simulink model "Model_6DOF_dk"  (R2022a)
settings: Solver=FixedStepAuto  StartTime=0.0  StopTime=Tf  FixedStep=0.05  RelTol=1e-3
InitFcn:
  | run;
StopFcn:
  | save('testdata')
values from neighbouring files (symbols this model uses):
  adap = 1    [run.m]    (also in testdata.mat)
  Ba_0 = [0 0 0 0 0 0]    [run.m]    (also in testdata.mat)
  Bb = 4418825.3321    [testdata.mat]
  Bv_0 = [-5.14444 0 0 0 0 0]    [run.m]    (also in testdata.mat)
  Bx_0 = [0 0 -12 0 0 0]    [run.m]    (also in testdata.mat)
  dA_BP1 = [0.00388591051125 0.00354364911083 0.00553040741788 0.00502167988714 0.0078585088908 0.00748424955325 0.0119232766011 0.0109054787122 0.0168329706434 0.016985509009 0.0156802934897 0.014556760782 ... (616 elements, 616x1)]    [testdata.mat]
  dA_BP2 = [0.00388594063171 0.00354357191533 0.00553040491113 0.00502170939051 0.00785855989083 0.00748435285791 0.0119232653011 0.0109054419481 0.0168329955973 0.0169854794658 0.015680230324 0.0145567225609 ... (616 elements, 616x1)]    [testdata.mat]
  dA_Hull = [0.896301676511 0.898896720864 0.884294141897 0.886832830172 0.870887902011 0.873360353662 0.856223658523 0.858613244346 0.840314828191 0.842595287849 0.823129385532 0.8253007603 ... (2914 elements, 2914x1)]    [testdata.mat]
  dA_PH = [0.00917454029683 0.00917454029683 0.00646521761836 0.00644666811643 0.011728531678 0.0107683420972 0.0165186720105 0.0100399866209 0.0121147162203 0.00917369783051 0.00917369783051 0.00646462373197 ... (550 elements, 550x1)]    [testdata.mat]
  dA_Sail = [0.08073747293 0.0655437895785 0.0678199581962 0.211496702297 0.185444652254 0.10949647106 0.0763960001413 0.0735864235671 0.0440728222699 0.281106392154 0.32735958292 0.104041938486 ... (564 elements, 564x1)]    [testdata.mat]
  dA_SProot = [0.0225345452169 0.0247277274893 0.0225345452169 0.0480467976325 0.0166447079844 0.0410754287554 0.0247277274893 0.0480467976325 0.0468898715351 0.0839833312794 0.0166447079844 0.0255016718 ... (904 elements, 904x1)]    [testdata.mat]
  dA_X1a = [0.0149621011817 0.0166706156701 0.0341149781095 0.0355915100668 0.0512235531199 0.0489176133683 0.0604458424392 0.0503279152264 0.0577124835488 0.0401555322121 0.044833653096 0.0251568218541 ... (200 elements, 200x1)]    [testdata.mat]
  dA_X1b = [0.0149621011817 0.0166706156701 0.0341149781095 0.0355915100668 0.0512235531199 0.0489176133683 0.0604458424392 0.0503279152264 0.0577124835488 0.0401555322121 0.044833653096 0.0251568218541 ... (200 elements, 200x1)]    [testdata.mat]
  dA_X2a = [0.0149620639393 0.0166705502855 0.0341150948266 0.0355913495849 0.051223110376 0.0489180393921 0.0604458270347 0.0503275686692 0.0577128112225 0.0401556683139 0.0448334591683 0.0251566482124 ... (200 elements, 200x1)]    [testdata.mat]
  dA_X2b = [0.0149620639393 0.0166705502855 0.0341150948266 0.0355913495849 0.051223110376 0.0489180393921 0.0604458270347 0.0503275686692 0.0577128112225 0.0401556683139 0.0448334591683 0.0251566482124 ... (200 elements, 200x1)]    [testdata.mat]
  dA_X3a = [0.0149621011817 0.0166706156701 0.0341149781095 0.0355915100668 0.0512235531199 0.0489176133683 0.0604458424392 0.0503279152264 0.0577124835488 0.0401555322121 0.044833653096 0.0251568218541 ... (200 elements, 200x1)]    [testdata.mat]
  dA_X3b = [0.0149621011817 0.0166706156701 0.0341149781095 0.0355915100668 0.0512235531199 0.0489176133683 0.0604458424392 0.0503279152264 0.0577124835488 0.0401555322121 0.044833653096 0.0251568218541 ... (200 elements, 200x1)]    [testdata.mat]
  dA_X4a = [0.0149621011817 0.0166706156701 0.0341149781095 0.0355915100668 0.0512235531199 0.0489176133683 0.0604458424392 0.0503279152264 0.0577124835488 0.0401555322121 0.044833653096 0.0251568218541 ... (200 elements, 200x1)]    [testdata.mat]
  dA_X4b = [0.0149621011817 0.0166706156701 0.0341149781095 0.0355915100668 0.0512235531199 0.0489176133683 0.0604458424392 0.0503279152264 0.0577124835488 0.0401555322121 0.044833653096 0.0251568218541 ... (200 elements, 200x1)]    [testdata.mat]
  Ixx = 52300000    [testdata.mat]
  Ixy = 0    [testdata.mat]
  Ixz = 0    [testdata.mat]
  Iyy = 1375000000    [testdata.mat]
  Iyz = 0    [testdata.mat]
  Izz = 1367000000    [testdata.mat]
  L1 =     [testdata.mat]
  Mb = 4418825.3321    [testdata.mat]
  n_BP1 = [-0.7747315 -0.03638153 -0.4095958 0 -0.1221389 0 -0.01670914 0 0.005209626 0 0.03404154 0 ... (1848 elements, 616x3)]    [testdata.mat]
  n_BP2 = [-0.774731517 -0.0363815315 -0.409595788 0 -0.122138903 0 -0.0167091396 0 0.00520962616 0 0.0340415388 0 ... (1848 elements, 616x3)]    [testdata.mat]
  n_Hull = [-3.334458e-05 -1.700098e-14 -3.354233e-05 -1.686235e-14 -3.289162e-05 -1.685701e-14 -3.291391e-05 -1.698144e-14 -3.338145e-05 -1.688959e-14 -3.29289e-05 -1.682536e-14 ... (8742 elements, 2914x3)]    [testdata.mat]
  n_PH = [0 0 0.01711651 0.01711627 0.2676807 0.2676804 0.7675173 0.7675174 0.9857236 0 0 0.01711456 ... (1650 elements, 550x3)]    [testdata.mat]
  n_Sail = [-0.05126832 -0.05168081 -0.0485872 -0.03288998 -0.03203588 -0.04435105 -0.04335441 -0.04419429 -0.05169604 0.01094904 0.01649325 -0.03825178 ... (1692 elements, 564x3)]    [testdata.mat]
  n_SProot = [-0.7837688 -0.7969784 -0.7837688 -0.79448 -0.280412 -0.3378876 -0.7969784 -0.79448 -0.7910827 -0.3483897 -0.280412 -0.2790298 ... (2712 elements, 904x3)]    [testdata.mat]
  n_X2a = [-0.283297986 -0.283136904 -0.283195704 -0.28313759 -0.2831586 -0.283137113 -0.28313911 -0.283136606 -0.283121586 -0.283136815 -0.283108413 -0.283138901 ... (600 elements, 200x3)]    [testdata.mat]
  n_X2b = [-0.283297986 -0.283136904 -0.283195704 -0.28313759 -0.2831586 -0.283137113 -0.28313911 -0.283136606 -0.283121586 -0.283136815 -0.283108413 -0.283138901 ... (600 elements, 200x3)]    [testdata.mat]
  n_X3a = [-0.283298 -0.2831369 -0.2831957 -0.2831376 -0.2831586 -0.2831371 -0.2831391 -0.2831366 -0.2831216 -0.2831368 -0.2831084 -0.2831389 ... (600 elements, 200x3)]    [testdata.mat]
  n_X4a = [-0.283298 -0.2831369 -0.2831957 -0.2831376 -0.2831586 -0.2831371 -0.2831391 -0.2831366 -0.2831216 -0.2831368 -0.2831084 -0.2831389 ... (600 elements, 200x3)]    [testdata.mat]
  n_X4b = [-0.283298 -0.2831369 -0.2831957 -0.2831376 -0.2831586 -0.2831371 -0.2831391 -0.2831366 -0.2831216 -0.2831368 -0.2831084 -0.2831389 ... (600 elements, 200x3)]    [testdata.mat]
  nt_BP1 = 616    [testdata.mat]
  nt_BP2 = 616    [testdata.mat]
  nt_Hull = 2914    [testdata.mat]
  nt_PH = 550    [testdata.mat]
  nt_Sail = 564    [testdata.mat]
  nt_SProot = 904    [testdata.mat]
  nt_X1a = 200    [testdata.mat]
  nt_X1b = 200    [testdata.mat]
  nt_X2a = 200    [testdata.mat]
  nt_X2b = 200    [testdata.mat]
  nt_X3a = 200    [testdata.mat]
  nt_X3b = 200    [testdata.mat]
  nt_X4a = 200    [testdata.mat]
  nt_X4b = 200    [testdata.mat]
  psi_ref = 0    [run.m]    (also in testdata.mat)
  Seastate = 0    [run.m]    (also in testdata.mat)
  Ts = 0.05    [run.m]    (also in testdata.mat)
  v_ref = Bv_0(1)    [run.m]    (also in testdata.mat = -5.14444)
  vt1_BP1 = [-11.0524049722 -10.9924120522 -10.9924120522 -10.8819663922 -10.8819663922 -10.7297166322 -10.7297166322 -10.5070632922 -10.5070632922 -10.1807245522 -10.1807245522 -9.8815181122 ... (1848 elements, 616x3)]    [testdata.mat]
  vt1_BP2 = [-11.0524048318 -10.9924111396 -10.9924111396 -10.8819658306 -10.8819658306 -10.7297157898 -10.7297157898 -10.5070637134 -10.5070637134 -10.1807238502 -10.1807238502 -9.8815188844 ... (1848 elements, 616x3)]    [testdata.mat]
  vt1_Hull = [3.5122487678 3.7304022878 5.2621803278 5.4863499878 6.9866994878 7.2167238278 8.6832650078 8.9189474678 10.3493567078 10.5904445678 11.9823842078 12.2286247478 ... (8742 elements, 2914x3)]    [testdata.mat]
  vt1_PH = [37.3342788278 37.3342788278 37.4268866678 37.4268866678 37.5892452278 37.5892452278 37.7549453078 37.7549453078 37.8074619278 37.3342788278 37.3342788278 37.4268866678 ... (1650 elements, 550x3)]    [testdata.mat]
  vt1_Sail = [-12.4909433722 -12.1578443722 -12.0399645322 -11.2138368922 -10.6240515922 -11.5111900522 -11.9364967522 -11.6561249722 -12.4909433722 -7.5732648922 -6.8453119522 -11.1890071522 ... (1692 elements, 564x3)]    [testdata.mat]
  vt1_SProot = [29.2099766678 29.1371231078 29.0494854278 29.2099766678 29.2862630078 29.4526510478 29.0494854278 29.1261368078 29.3369263478 29.5706712878 29.0494854278 29.3857364078 ... (2712 elements, 904x3)]    [testdata.mat]
  vt1_X1a = [29.3961751478 29.4776282078 29.4776282078 29.7060309278 29.7060309278 30.0693861278 30.0693861278 30.5458756478 30.5458756478 31.0830460478 31.0830460478 31.6023926678 ... (600 elements, 200x3)]    [testdata.mat]
  vt1_X1b = [29.6638337078 29.6638337078 29.9620713878 29.9620713878 30.3181187678 30.3181187678 30.7116389078 30.7116389078 31.1104380878 31.1104380878 31.4810519678 31.4810519678 ... (600 elements, 200x3)]    [testdata.mat]
  vt1_X2a = [29.3961767624 29.4776272952 29.4776272952 29.7060326828 29.7060326828 30.0693842324 30.0693842324 30.5458736822 30.5458736822 31.083047171 31.083047171 31.6023916148 ... (600 elements, 200x3)]    [testdata.mat]
  vt1_X2b = [29.6638345502 29.6638345502 29.9620708964 29.9620708964 30.3181168022 30.3181168022 30.7116409436 30.7116409436 31.1104372454 31.1104372454 31.4810526698 31.4810526698 ... (600 elements, 200x3)]    [testdata.mat]
  vt1_X3a = [29.3961751478 29.4776282078 29.4776282078 29.7060309278 29.7060309278 30.0693861278 30.0693861278 30.5458756478 30.5458756478 31.0830460478 31.0830460478 31.6023926678 ... (600 elements, 200x3)]    [testdata.mat]
  vt1_X3b = [29.6638337078 29.6638337078 29.9620713878 29.9620713878 30.3181187678 30.3181187678 30.7116389078 30.7116389078 31.1104380878 31.1104380878 31.4810519678 31.4810519678 ... (600 elements, 200x3)]    [testdata.mat]
  vt1_X4a = [29.6638337078 29.6638337078 29.9620713878 29.9620713878 30.3181187678 30.3181187678 30.7116389078 30.7116389078 31.1104380878 31.1104380878 31.4810519678 31.4810519678 ... (600 elements, 200x3)]    [testdata.mat]
  vt1_X4b = [29.3961751478 29.4776282078 29.4776282078 29.7060309278 29.7060309278 30.0693861278 30.0693861278 30.5458756478 30.5458756478 31.0830460478 31.0830460478 31.6023926678 ... (600 elements, 200x3)]    [testdata.mat]
  vt2_BP1 = [-10.9924120522 -10.9494777322 -10.8819663922 -10.8505308322 -10.7297166322 -10.7112259522 -10.5070632922 -10.4997203722 -10.1807245522 -10.1757543922 -9.8815181122 -9.8813004922 ... (1848 elements, 616x3)]    [testdata.mat]
  vt2_BP2 = [-11.0294626294 -11.0294626294 -10.9494786448 -10.9494786448 -10.8505316746 -10.8505316746 -10.7112256012 -10.7112256012 -10.499720302 -10.499720302 -10.1757550942 -10.1757550942 ... (1848 elements, 616x3)]    [testdata.mat]
  vt2_Hull = [1.9517168078 1.9517168078 3.7304022878 3.7304022878 5.4863499878 5.4863499878 7.2167238278 7.2167238278 8.9189474678 8.9189474678 10.5904445678 10.5904445678 ... (8742 elements, 2914x3)]    [testdata.mat]
  vt2_PH = [37.2028433678 37.2028433678 37.3342788278 37.4268866678 37.4268866678 37.5892452278 37.5892452278 37.7549453078 37.7549453078 37.2028433678 37.2028433678 37.3342788278 ... (1650 elements, 550x3)]    [testdata.mat]
  vt2_Sail = [-12.0399645322 -12.0399645322 -11.9364967522 -10.7084881522 -10.7084881522 -12.0399645322 -12.0399645322 -11.9364967522 -12.3734566522 -7.7110323922 -7.7110323922 -11.6561249722 ... (1692 elements, 564x3)]    [testdata.mat]
  vt2_SProot = [29.0494854278 29.0494854278 29.2099766678 29.1261368078 29.0494854278 29.1371231078 29.1371231078 29.2099766678 29.1261368078 29.2099766678 29.2862630078 29.2862630078 ... (2712 elements, 904x3)]    [testdata.mat]
  vt2_X1a = [29.4776282078 29.9620713878 29.7060309278 30.3181187678 30.0693861278 30.7116389078 30.5458756478 31.1104380878 31.0830460478 31.4810519678 31.6023926678 31.7970362078 ... (600 elements, 200x3)]    [testdata.mat]
  vt2_X1b = [29.4776282078 29.9620713878 29.7060309278 30.3181187678 30.0693861278 30.7116389078 30.5458756478 31.1104380878 31.0830460478 31.4810519678 31.6023926678 31.7970362078 ... (600 elements, 200x3)]    [testdata.mat]
  vt2_X2a = [29.6638345502 29.6638345502 29.9620708964 29.9620708964 30.3181168022 30.3181168022 30.7116409436 30.7116409436 31.1104372454 31.1104372454 31.4810526698 31.4810526698 ... (600 elements, 200x3)]    [testdata.mat]
  vt2_X2b = [29.3961767624 29.4776272952 29.4776272952 29.7060326828 29.7060326828 30.0693842324 30.0693842324 30.5458736822 30.5458736822 31.083047171 31.083047171 31.6023916148 ... (600 elements, 200x3)]    [testdata.mat]
  vt2_X3a = [29.4776282078 29.9620713878 29.7060309278 30.3181187678 30.0693861278 30.7116389078 30.5458756478 31.1104380878 31.0830460478 31.4810519678 31.6023926678 31.7970362078 ... (600 elements, 200x3)]    [testdata.mat]
  vt2_X3b = [29.4776282078 29.9620713878 29.7060309278 30.3181187678 30.0693861278 30.7116389078 30.5458756478 31.1104380878 31.0830460478 31.4810519678 31.6023926678 31.7970362078 ... (600 elements, 200x3)]    [testdata.mat]
  vt2_X4a = [29.4776282078 29.9620713878 29.7060309278 30.3181187678 30.0693861278 30.7116389078 30.5458756478 31.1104380878 31.0830460478 31.4810519678 31.6023926678 31.7970362078 ... (600 elements, 200x3)]    [testdata.mat]
  vt2_X4b = [29.4776282078 29.9620713878 29.7060309278 30.3181187678 30.0693861278 30.7116389078 30.5458756478 31.1104380878 31.0830460478 31.4810519678 31.6023926678 31.7970362078 ... (600 elements, 200x3)]    [testdata.mat]
  vt3_BP1 = [-11.0294636122 -11.0294636122 -10.9494777322 -10.9494777322 -10.8505308322 -10.8505308322 -10.7112259522 -10.7112259522 -10.4997203722 -10.4997203722 -10.1757543922 -10.1757543922 ... (1848 elements, 616x3)]    [testdata.mat]
  vt3_BP2 = [-10.9924111396 -10.9494786448 -10.8819658306 -10.8505316746 -10.7297157898 -10.7112256012 -10.5070637134 -10.499720302 -10.1807238502 -10.1757550942 -9.8815188844 -9.8813013346 ... (1848 elements, 616x3)]    [testdata.mat]
  vt3_Hull = [1.7397198278 3.5122487678 3.5122487678 5.2621803278 5.2621803278 6.9866994878 6.9866994878 8.6832650078 8.6832650078 10.3493567078 10.3493567078 11.9823842078 ... (8742 elements, 2914x3)]    [testdata.mat]
  vt3_PH = [37.2028433678 37.3342788278 37.3342788278 37.3342788278 37.4268866678 37.4268866678 37.5892452278 37.5892452278 37.7549453078 37.2028433678 37.3342788278 37.3342788278 ... (1650 elements, 550x3)]    [testdata.mat]
  vt3_Sail = [-12.3734566522 -12.4909433722 -12.3734566522 -11.5111900522 -11.2138368922 -11.7698559922 -11.5111900522 -11.5111900522 -12.1578443722 -8.3109054322 -7.5732648922 -11.5111900522 ... (1692 elements, 564x3)]    [testdata.mat]
  vt3_SProot = [29.1261368078 29.2099766678 29.1261368078 29.3369263478 29.1371231078 29.2099766678 29.2099766678 29.3369263478 29.2548344678 29.3369263478 29.1371231078 29.1371231078 ... (2712 elements, 904x3)]    [testdata.mat]
  vt3_X1a = [29.6638337078 29.6638337078 29.9620713878 29.9620713878 30.3181187678 30.3181187678 30.7116389078 30.7116389078 31.1104380878 31.1104380878 31.4810519678 31.4810519678 ... (600 elements, 200x3)]    [testdata.mat]
  vt3_X1b = [29.3961751478 29.4776282078 29.4776282078 29.7060309278 29.7060309278 30.0693861278 30.0693861278 30.5458756478 30.5458756478 31.0830460478 31.0830460478 31.6023926678 ... (600 elements, 200x3)]    [testdata.mat]
  vt3_X2a = [29.4776272952 29.9620708964 29.7060326828 30.3181168022 30.0693842324 30.7116409436 30.5458736822 31.1104372454 31.083047171 31.4810526698 31.6023916148 31.7970343826 ... (600 elements, 200x3)]    [testdata.mat]
  vt3_X2b = [29.4776272952 29.9620708964 29.7060326828 30.3181168022 30.0693842324 30.7116409436 30.5458736822 31.1104372454 31.083047171 31.4810526698 31.6023916148 31.7970343826 ... (600 elements, 200x3)]    [testdata.mat]
  vt3_X3a = [29.6638337078 29.6638337078 29.9620713878 29.9620713878 30.3181187678 30.3181187678 30.7116389078 30.7116389078 31.1104380878 31.1104380878 31.4810519678 31.4810519678 ... (600 elements, 200x3)]    [testdata.mat]
  vt3_X3b = [29.3961751478 29.4776282078 29.4776282078 29.7060309278 29.7060309278 30.0693861278 30.0693861278 30.5458756478 30.5458756478 31.0830460478 31.0830460478 31.6023926678 ... (600 elements, 200x3)]    [testdata.mat]
  vt3_X4a = [29.3961751478 29.4776282078 29.4776282078 29.7060309278 29.7060309278 30.0693861278 30.0693861278 30.5458756478 30.5458756478 31.0830460478 31.0830460478 31.6023926678 ... (600 elements, 200x3)]    [testdata.mat]
  vt3_X4b = [29.6638337078 29.6638337078 29.9620713878 29.9620713878 30.3181187678 30.3181187678 30.7116389078 30.7116389078 31.1104380878 31.1104380878 31.4810519678 31.4810519678 ... (600 elements, 200x3)]    [testdata.mat]
  Xb = 0    [testdata.mat]
  Xcg = [32.3287332922 0 0]    [testdata.mat]
  Xg = 0    [testdata.mat]
  Yb = 0    [testdata.mat]
  Yg = 0    [testdata.mat]
  z_ref = Bx_0(3)    [run.m]    (also in testdata.mat = -12)
  Zb = 0.4406    [testdata.mat]
  Zg = 0    [testdata.mat]
libraries: simulink x8
(part 4 of 8)

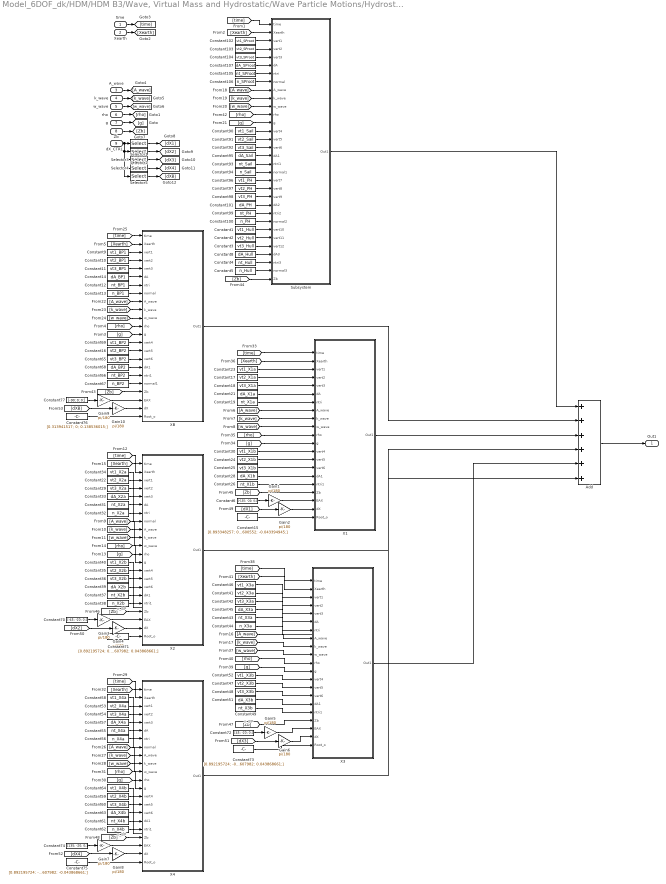
== system Model_6DOF_dk/HDM/HDM B3/Wave, Virtual Mass and Hydrostatic/Wave Particle Motions/Hydrostatic Forces and Moments ==
  note: n_BP
  note: n_BP
  note: n_BP
  time : Inport
  Xearth : Inport  Port=2
  A_wave : Inport  Port=3
  k_wave : Inport  Port=4
  w_wave : Inport  Port=5
  rho : Inport  Port=6
  g : Inport  Port=7
  Zb : Inport  Port=8
  dX_CTRL : Inport  Port=9
  Add : Sum  Inputs=6
  Constant1 : Constant  Value=vt1_Hull
  Constant10 : Constant  Value=vt2_BP1
  Constant100 : Constant  Value=n_PH
  Constant101 : Constant  Value=dA_PH
  Constant102 : Constant  Value=vt1_SProot
  Constant103 : Constant  Value=vt2_SProot
  Constant104 : Constant  Value=vt3_SProot
  Constant105 : Constant  Value=nt_SProot
  Constant106 : Constant  Value=n_SProot
  Constant107 : Constant  Value=dA_SProot
  Constant11 : Constant  Value=vt3_BP1
  Constant12 : Constant  Value=nt_BP1
  Constant13 : Constant  Value=n_BP1
  Constant14 : Constant  Value=dA_BP1
  Constant15 : Constant  Value=|
      | [0.893348257;
      | 0.043600552;
      | -0.043394945;]
  Constant16 : Constant  Value=vt2_BP2
  Constant17 : Constant  Value=vt2_X1a
  Constant18 : Constant  Value=vt3_X1a
  Constant19 : Constant  Value=nt_X1a
  Constant2 : Constant  Value=vt2_Hull
  Constant21 : Constant  Value=dA_X1a
  Constant22 : Constant  Value=vt2_X2a
  Constant23 : Constant  Value=vt1_X1a
  Constant24 : Constant  Value=vt2_X1b
  Constant25 : Constant  Value=vt3_X1b
  Constant26 : Constant  Value=nt_X1b
  Constant28 : Constant  Value=dA_X1b
  Constant29 : Constant  Value=vt3_X2a
  Constant3 : Constant  Value=vt3_Hull
  Constant30 : Constant  Value=vt1_X1b
  Constant31 : Constant  Value=nt_X2a
  Constant32 : Constant  Value=n_X2a
  Constant33 : Constant  Value=dA_X2a
  Constant34 : Constant  Value=vt1_X2a
  Constant35 : Constant  Value=vt2_X2b
  Constant36 : Constant  Value=vt3_X2b
  Constant37 : Constant  Value=nt_X2b
  Constant38 : Constant  Value=n_X2b
  Constant39 : Constant  Value=dA_X2b
  Constant4 : Constant  Value=nt_Hull
  Constant40 : Constant  Value=vt1_X2b
  Constant41 : Constant  Value=vt2_X3a
  Constant42 : Constant  Value=vt3_X3a
  Constant43 : Constant  Value=nt_X3a
  Constant44 : Constant  Value=n_X3a
  Constant45 : Constant  Value=dA_X3a
  Constant46 : Constant  Value=vt1_X3a
  Constant47 : Constant  Value=vt2_X3b
  Constant48 : Constant  Value=vt3_X3b
  Constant49 : Constant  Value=nt_X3b
  Constant5 : Constant  Value=n_Hull
  Constant51 : Constant  Value=dA_X3b
  Constant52 : Constant  Value=vt1_X3b
  Constant53 : Constant  Value=vt2_X4a
  Constant54 : Constant  Value=vt3_X4a
  Constant55 : Constant  Value=nt_X4a
  Constant56 : Constant  Value=n_X4a
  Constant57 : Constant  Value=dA_X4a
  Constant58 : Constant  Value=vt1_X4a
  Constant59 : Constant  Value=vt2_X4b
  Constant6 : Constant  Value=[-135; -20; 0;]
  Constant60 : Constant  Value=vt3_X4b
  Constant61 : Constant  Value=nt_X4b
  Constant62 : Constant  Value=n_X4b
  Constant63 : Constant  Value=dA_X4b
  Constant64 : Constant  Value=vt1_X4b
  Constant65 : Constant  Value=vt3_BP2
  Constant66 : Constant  Value=nt_BP2
  Constant67 : Constant  Value=n_BP2
  Constant68 : Constant  Value=dA_BP2
  Constant69 : Constant  Value=vt1_BP2
  Constant70 : Constant  Value=[-45; -20; 0;]
  Constant71 : Constant  Value=|
      | [0.892195724;
      | 0.043607982;
      | 0.043868661;]
  Constant72 : Constant  Value=[45; -20; 0;]
  Constant73 : Constant  Value=|
      | [0.892195724;
      | -0.043607982;
      | 0.043868661;]
  Constant74 : Constant  Value=[135; -20; 0;]
  Constant75 : Constant  Value=|
      | [0.892195724;
      | -0.043607982;
      | -0.043868661;]
  Constant76 : Constant  Value=|
      | [0.313941517;
      | 0;
      | 0.138536015;]
  Constant77 : Constant  Value=[-90; 0; 0;]
  Constant8 : Constant  Value=dA_Hull
  Constant9 : Constant  Value=vt1_BP1
  Constant90 : Constant  Value=vt1_Sail
  Constant91 : Constant  Value=vt2_Sail
  Constant92 : Constant  Value=vt3_Sail
  Constant93 : Constant  Value=nt_Sail
  Constant94 : Constant  Value=n_Sail
  Constant95 : Constant  Value=dA_Sail
  Constant96 : Constant  Value=vt1_PH
  Constant97 : Constant  Value=vt2_PH
  Constant98 : Constant  Value=vt3_PH
  Constant99 : Constant  Value=nt_PH
  Gain{1..10} (10 alike) : Gain  Gain=pi/180
  Selector1 : Selector  InputPortWidth=5  IndexOptions=Index vector (dialog)  Indices=1  OutputSizes=1
  Selector2 : Selector  InputPortWidth=5  IndexOptions=Index vector (dialog)  Indices=2  OutputSizes=1
  Selector3 : Selector  InputPortWidth=5  IndexOptions=Index vector (dialog)  Indices=3  OutputSizes=1
  Selector4 : Selector  InputPortWidth=5  IndexOptions=Index vector (dialog)  Indices=4  OutputSizes=1
  Selector5 : Selector  InputPortWidth=5  IndexOptions=Index vector (dialog)  Indices=5  OutputSizes=1
  Subsystem : Subsystem
  X1 : Subsystem
  X2 : Subsystem
  X3 : Subsystem
  X4 : Subsystem
  XB : Subsystem
  Out1 : Outport
  wires:
  Subsystem/1(Out1) -> Add/1
  XB/1(Out1) -> Add/2
  X1/1(Out1) -> Add/3
  X2/1(Out1) -> Add/4
  X3/1(Out1) -> Add/5
  X4/1(Out1) -> Add/6
  Gain10/1 -> XB/22(dX)
  Constant76/1 -> XB/23(Root_o)
  [dXB] -> Gain10/1
  Gain9/1 -> XB/21(EAX)
  Constant77/1 -> Gain9/1
  Gain8/1 -> X4/21(dX)
  [dX4] -> Gain8/1
  Constant74/1 -> Gain7/1
  Gain7/1 -> X4/20(EAX)
  Constant75/1 -> X4/22(Root_o)
  Constant73/1 -> X3/21(Root_o)
  Gain6/1 -> X3/20(dX)
  Constant72/1 -> Gain5/1
  [dX3] -> Gain6/1
  Gain5/1 -> X3/19(EAX)
  Constant71/1 -> X2/22(Root_o)
  Gain4/1 -> X2/21(dX)
  [dX2] -> Gain4/1
  Gain3/1 -> X2/20(EAX)
  Constant70/1 -> Gain3/1
  Constant15/1 -> X1/21(Root_o)
  Gain2/1 -> X1/20(dX)
  [dX1] -> Gain2/1
  Selector5/1 -> [dXB]
  Selector4/1 -> [dX4]
  Selector3/1 -> [dX3]
  Selector2/1 -> [dX2]
  Selector1/1 -> [dX1]
  dX_CTRL/1 -> Selector1/1, Selector4/1, Selector5/1, Selector3/1, Selector2/1
  Gain1/1 -> X1/19(EAX)
  Constant6/1 -> Gain1/1
  Zb/1 -> [Zb]
  [A_wave] -> X3/8(A_wave)
  Constant5/1 -> Subsystem/31(normal3)
  Constant58/1 -> X4/3(vert1)
  Constant42/1 -> X3/5(vert3)
  [g] -> XB/13(g)
  Constant3/1 -> Subsystem/28(vert12)
  Constant103/1 -> Subsystem/4(vert2)
  Add/1 -> Out1/1
  [A_wave] -> Subsystem/9(A_wave)
  Constant10/1 -> XB/4(vert2)
  [time] -> X4/1(time)
  [k_wave] -> X4/10(k_wave)
  Constant38/1 -> ?
  Constant54/1 -> X4/5(vert3)
  Constant66/1 -> XB/18(ntri1)
  Constant2/1 -> Subsystem/27(vert11)
  Constant97/1 -> Subsystem/21(vert8)
  Constant64/1 -> X4/14(vert4)
  [Xearth] -> X4/2(Xearth)
  Constant29/1 -> X2/5(vert3)
  Constant36/1 -> X2/16(vert6)
  Constant96/1 -> Subsystem/20(vert7)
  Constant90/1 -> Subsystem/14(vert4)
  Constant21/1 -> X1/6(dA)
  [w_wave] -> X2/11(w_wave)
  Constant31/1 -> X2/7(ntri)
  Constant1/1 -> Subsystem/26(vert10)
  [time] -> X1/1(time)
  Constant91/1 -> Subsystem/15(vert5)
  [rho] -> X1/11(rho)
  [time] -> X2/1(time)
  Constant30/1 -> X1/13(vert4)
  Constant92/1 -> Subsystem/16(vert6)
  Constant100/1 -> Subsystem/25(normal2)
  [w_wave] -> X1/10(w_wave)
  [g] -> X3/12(g)
  Constant12/1 -> XB/7(ntri)
  Constant24/1 -> X1/14(vert5)
  Constant56/1 -> X4/8(normal)
  Constant26/1 -> X1/17(ntri1)
  [A_wave] -> XB/9(A_wave)
  Constant62/1 -> ?
  Constant9/1 -> XB/3(vert1)
  Constant23/1 -> X1/3(vert1)
  Constant46/1 -> X3/3(vert1)
  Constant68/1 -> XB/17(dA1)
  [k_wave] -> XB/10(k_wave)
  Constant17/1 -> X1/4(vert2)
  [A_wave] -> X2/9(A_wave)
  [k_wave] -> X3/9(k_wave)
  Constant43/1 -> X3/7(ntri)
  Constant69/1 -> XB/14(vert4)
  Constant13/1 -> XB/8(normal)
  Constant104/1 -> Subsystem/5(vert3)
  Constant65/1 -> XB/16(vert6)
  [Zb] -> Subsystem/32(Zb)
  Constant67/1 -> XB/19(normal1)
  Constant25/1 -> X1/15(vert6)
  [Xearth] -> X3/2(Xearth)
  Constant14/1 -> XB/6(dA)
  Constant52/1 -> X3/13(vert4)
  Constant51/1 -> X3/16(dA1)
  Constant59/1 -> X4/15(vert5)
  Constant4/1 -> Subsystem/30(ntri3)
  [rho] -> XB/12(rho)
  [time] -> XB/1(time)
  [Xearth] -> X2/2(Xearth)
  [w_wave] -> XB/11(w_wave)
  Constant53/1 -> X4/4(vert2)
  [k_wave] -> X1/9(k_wave)
  Constant44/1 -> ?
  [w_wave] -> X4/11(w_wave)
  Constant47/1 -> X3/14(vert5)
  Constant32/1 -> X2/8(normal)
  Constant39/1 -> X2/17(dA1)
  Constant35/1 -> X2/15(vert5)
  [g] -> X1/12(g)
  Constant18/1 -> X1/5(vert3)
  Constant40/1 -> X2/14(vert4)
  Constant45/1 -> X3/6(dA)
  Constant55/1 -> X4/7(ntri)
  [rho] -> X3/11(rho)
  [rho] -> X2/12(rho)
  [Xearth] -> XB/2(Xearth)
  Constant49/1 -> X3/17(ntri1)
  Constant22/1 -> X2/4(vert2)
  [k_wave] -> X2/10(k_wave)
  Constant41/1 -> X3/4(vert2)
  [A_wave] -> X1/8(A_wave)
  Constant63/1 -> X4/17(dA1)
  Constant34/1 -> X2/3(vert1)
  Constant11/1 -> XB/5(vert3)
  [g] -> X4/13(g)
  Constant105/1 -> Subsystem/7(ntri)
  Constant107/1 -> Subsystem/6(dA)
  [Xearth] -> Subsystem/2(Xearth)
  Constant106/1 -> Subsystem/8(normal)
  Constant102/1 -> Subsystem/3(vert1)
  [g] -> Subsystem/13(g)
  Constant19/1 -> X1/7(ntri)
  [k_wave] -> Subsystem/10(k_wave)
  Constant60/1 -> X4/16(vert6)
  [rho] -> Subsystem/12(rho)
  Constant48/1 -> X3/15(vert6)
  [time] -> Subsystem/1(time)
  [rho] -> X4/12(rho)
  Constant33/1 -> X2/6(dA)
  [A_wave] -> X4/9(A_wave)
  Constant95/1 -> Subsystem/17(dA1)
  Constant8/1 -> Subsystem/29(dA3)
  [w_wave] -> X3/10(w_wave)
  Constant28/1 -> X1/16(dA1)
  [g] -> X2/13(g)
  Constant93/1 -> Subsystem/18(ntri1)
  [w_wave] -> Subsystem/11(w_wave)
  [Xearth] -> X1/2(Xearth)
  [time] -> X3/1(time)
  [Zb] -> XB/20(Zb)
  Constant37/1 -> X2/18(ntri1)
  Constant99/1 -> Subsystem/24(ntri2)
  Constant98/1 -> Subsystem/22(vert9)
  [Zb] -> X2/19(Zb)
  [Zb] -> X1/18(Zb)
  Constant16/1 -> XB/15(vert5)
  Constant101/1 -> Subsystem/23(dA2)
  [Zb] -> X3/18(Zb)
  [Zb] -> X4/19(Zb)
  Constant57/1 -> X4/6(dA)
  Constant61/1 -> X4/18(ntri1)
  Constant94/1 -> Subsystem/19(normal1)
  g/1 -> [g]
  rho/1 -> [rho]
  w_wave/1 -> [w_wave]
  k_wave/1 -> [k_wave]
  A_wave/1 -> [A_wave]
  Xearth/1 -> [Xearth]
  time/1 -> [time]

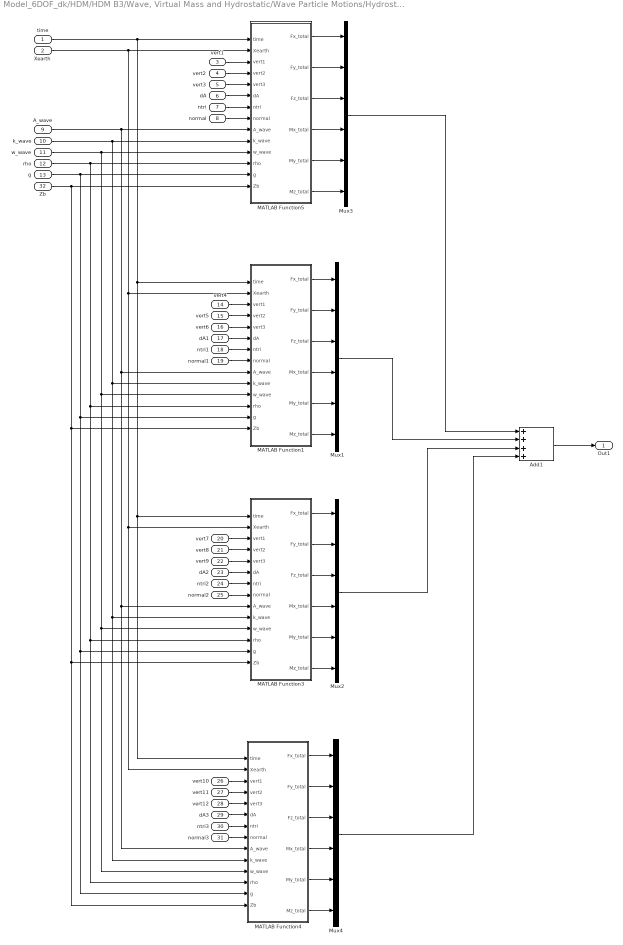
== system Model_6DOF_dk/HDM/HDM B3/Wave, Virtual Mass and Hydrostatic/Wave Particle Motions/Hydrostatic Forces and Moments/Subsystem ==
  time : Inport
  Xearth : Inport  Port=2
  vert1 : Inport  Port=3
  vert2 : Inport  Port=4
  vert3 : Inport  Port=5
  dA : Inport  Port=6
  ntri : Inport  Port=7
  normal : Inport  Port=8
  A_wave : Inport  Port=9
  k_wave : Inport  Port=10
  w_wave : Inport  Port=11
  rho : Inport  Port=12
  g : Inport  Port=13
  vert4 : Inport  Port=14
  vert5 : Inport  Port=15
  vert6 : Inport  Port=16
  dA1 : Inport  Port=17
  ntri1 : Inport  Port=18
  normal1 : Inport  Port=19
  vert7 : Inport  Port=20
  vert8 : Inport  Port=21
  vert9 : Inport  Port=22
  dA2 : Inport  Port=23
  ntri2 : Inport  Port=24
  normal2 : Inport  Port=25
  vert10 : Inport  Port=26
  vert11 : Inport  Port=27
  vert12 : Inport  Port=28
  dA3 : Inport  Port=29
  ntri3 : Inport  Port=30
  normal3 : Inport  Port=31
  Zb : Inport  Port=32
  Add1 : Sum  Inputs=4
  MATLAB Function1 : MATLAB Function  TreatAsAtomicUnit=on
  MATLAB Function3 : MATLAB Function  TreatAsAtomicUnit=on
  MATLAB Function4 : MATLAB Function  TreatAsAtomicUnit=on
  MATLAB Function5 : MATLAB Function  TreatAsAtomicUnit=on
  Mux{1..4} (4 alike) : Mux  Inputs=6
  Out1 : Outport
  wires:
  Mux4/1 -> Add1/4
  MATLAB Function4/5(My_total) -> Mux4/5
  MATLAB Function4/4(Mx_total) -> Mux4/4
  MATLAB Function4/3(Fz_total) -> Mux4/3
  MATLAB Function4/2(Fy_total) -> Mux4/2
  MATLAB Function4/1(Fx_total) -> Mux4/1
  MATLAB Function4/6(Mz_total) -> Mux4/6
  MATLAB Function3/6(Mz_total) -> Mux2/6
  MATLAB Function3/1(Fx_total) -> Mux2/1
  MATLAB Function3/2(Fy_total) -> Mux2/2
  MATLAB Function3/3(Fz_total) -> Mux2/3
  MATLAB Function3/4(Mx_total) -> Mux2/4
  MATLAB Function3/5(My_total) -> Mux2/5
  MATLAB Function1/5(My_total) -> Mux1/5
  MATLAB Function1/4(Mx_total) -> Mux1/4
  MATLAB Function1/3(Fz_total) -> Mux1/3
  MATLAB Function1/2(Fy_total) -> Mux1/2
  MATLAB Function1/1(Fx_total) -> Mux1/1
  Mux1/1 -> Add1/2
  MATLAB Function1/6(Mz_total) -> Mux1/6
  Mux2/1 -> Add1/3
  Zb/1 -> MATLAB Function4/14(Zb), MATLAB Function3/14(Zb), MATLAB Function1/14(Zb), MATLAB Function5/14(Zb)
  vert8/1 -> MATLAB Function3/4(vert2)
  vert1/1 -> MATLAB Function5/3(vert1)
  vert10/1 -> MATLAB Function4/3(vert1)
  dA1/1 -> MATLAB Function1/6(dA)
  normal2/1 -> MATLAB Function3/8(normal)
  vert3/1 -> MATLAB Function5/5(vert3)
  vert6/1 -> MATLAB Function1/5(vert3)
  Add1/1 -> Out1/1
  vert2/1 -> MATLAB Function5/4(vert2)
  dA3/1 -> MATLAB Function4/6(dA)
  ntri3/1 -> MATLAB Function4/7(ntri)
  ntri2/1 -> MATLAB Function3/7(ntri)
  vert11/1 -> MATLAB Function4/4(vert2)
  MATLAB Function5/6(Mz_total) -> Mux3/6
  dA/1 -> MATLAB Function5/6(dA)
  normal/1 -> MATLAB Function5/8(normal)
  vert9/1 -> MATLAB Function3/5(vert3)
  vert4/1 -> MATLAB Function1/3(vert1)
  normal3/1 -> MATLAB Function4/8(normal)
  vert12/1 -> MATLAB Function4/5(vert3)
  MATLAB Function5/1(Fx_total) -> Mux3/1
  dA2/1 -> MATLAB Function3/6(dA)
  g/1 -> MATLAB Function3/13(g), MATLAB Function4/13(g), MATLAB Function1/13(g), MATLAB Function5/13(g)
  ntri/1 -> MATLAB Function5/7(ntri)
  MATLAB Function5/2(Fy_total) -> Mux3/2
  w_wave/1 -> MATLAB Function3/11(w_wave), MATLAB Function4/11(w_wave), MATLAB Function1/11(w_wave), MATLAB Function5/11(w_wave)
  k_wave/1 -> MATLAB Function3/10(k_wave), MATLAB Function4/10(k_wave), MATLAB Function1/10(k_wave), MATLAB Function5/10(k_wave)
  MATLAB Function5/3(Fz_total) -> Mux3/3
  A_wave/1 -> MATLAB Function3/9(A_wave), MATLAB Function4/9(A_wave), MATLAB Function1/9(A_wave), MATLAB Function5/9(A_wave)
  normal1/1 -> MATLAB Function1/8(normal)
  Mux3/1 -> Add1/1
  MATLAB Function5/4(Mx_total) -> Mux3/4
  vert7/1 -> MATLAB Function3/3(vert1)
  Xearth/1 -> MATLAB Function1/2(Xearth), MATLAB Function3/2(Xearth), MATLAB Function4/2(Xearth), MATLAB Function5/2(Xearth)
  time/1 -> MATLAB Function3/1(time), MATLAB Function4/1(time), MATLAB Function1/1(time), MATLAB Function5/1(time)
  MATLAB Function5/5(My_total) -> Mux3/5
  vert5/1 -> MATLAB Function1/4(vert2)
  rho/1 -> MATLAB Function3/12(rho), MATLAB Function4/12(rho), MATLAB Function1/12(rho), MATLAB Function5/12(rho)
  ntri1/1 -> MATLAB Function1/7(ntri)

== system Model_6DOF_dk/HDM/HDM B3/Wave, Virtual Mass and Hydrostatic/Wave Particle Motions/Hydrostatic Forces and Moments/X1 ==
  time : Inport
  Xearth : Inport  Port=2
  vert1 : Inport  Port=3
  vert2 : Inport  Port=4
  vert3 : Inport  Port=5
  dA : Inport  Port=6
  ntri : Inport  Port=7
  A_wave : Inport  Port=8
  k_wave : Inport  Port=9
  w_wave : Inport  Port=10
  rho : Inport  Port=11
  g : Inport  Port=12
  vert4 : Inport  Port=13
  vert5 : Inport  Port=14
  vert6 : Inport  Port=15
  dA1 : Inport  Port=16
  ntri1 : Inport  Port=17
  Zb : Inport  Port=18
  EAX : Inport  Port=19
  dX : Inport  Port=20
  Root_o : Inport  Port=21
  Add1 : Sum
  CG : Constant  Value=[32.3114; 0; 0;]
  MATLAB Function1 : MATLAB Function  TreatAsAtomicUnit=on
  MATLAB Function4 : MATLAB Function  TreatAsAtomicUnit=on
  Mux1 : Mux  Inputs=6
  Mux2 : Mux  Inputs=6
  Out1 : Outport
  wires:
  MATLAB Function1/6(Mz_total) -> Mux1/6
  MATLAB Function1/5(My_total) -> Mux1/5
  CG/1 -> MATLAB Function4/17(xcg), MATLAB Function1/17(xcg)
  Root_o/1 -> MATLAB Function4/16(origin), MATLAB Function1/16(origin)
  dX/1 -> MATLAB Function1/15(dX), MATLAB Function4/15(dX)
  EAX/1 -> MATLAB Function4/14(EAX), MATLAB Function1/14(EAX)
  MATLAB Function4/3(Fz_total) -> Mux2/3
  MATLAB Function4/4(Mx_total) -> Mux2/4
  w_wave/1 -> MATLAB Function4/10(w_wave), MATLAB Function1/10(w_wave)
  MATLAB Function1/2(Fy_total) -> Mux1/2
  Xearth/1 -> MATLAB Function1/2(Xearth), MATLAB Function4/2(Xearth)
  rho/1 -> MATLAB Function4/11(rho), MATLAB Function1/11(rho)
  A_wave/1 -> MATLAB Function4/8(A_wave), MATLAB Function1/8(A_wave)
  MATLAB Function1/4(Mx_total) -> Mux1/4
  MATLAB Function4/1(Fx_total) -> Mux2/1
  MATLAB Function1/1(Fx_total) -> Mux1/1
  Add1/1 -> Out1/1
  MATLAB Function1/3(Fz_total) -> Mux1/3
  MATLAB Function4/5(My_total) -> Mux2/5
  dA/1 -> MATLAB Function4/6(dA)
  k_wave/1 -> MATLAB Function1/9(k_wave), MATLAB Function4/9(k_wave)
  g/1 -> MATLAB Function4/12(g), MATLAB Function1/12(g)
  MATLAB Function4/6(Mz_total) -> Mux2/6
  MATLAB Function4/2(Fy_total) -> Mux2/2
  Mux2/1 -> Add1/1
  vert3/1 -> MATLAB Function4/5(vert3)
  Mux1/1 -> Add1/2
  vert1/1 -> MATLAB Function4/3(vert1)
  time/1 -> MATLAB Function1/1(time), MATLAB Function4/1(time)
  ntri/1 -> MATLAB Function4/7(ntri)
  vert2/1 -> MATLAB Function4/4(vert2)
  Zb/1 -> MATLAB Function4/13(Zb), MATLAB Function1/13(Zb)
  vert4/1 -> MATLAB Function1/3(vert1)
  vert5/1 -> MATLAB Function1/4(vert2)
  vert6/1 -> MATLAB Function1/5(vert3)
  dA1/1 -> MATLAB Function1/6(dA)
  ntri1/1 -> MATLAB Function1/7(ntri)

== system Model_6DOF_dk/HDM/HDM B3/Wave, Virtual Mass and Hydrostatic/Wave Particle Motions/Hydrostatic Forces and Moments/X2 ==
  time : Inport
  Xearth : Inport  Port=2
  vert1 : Inport  Port=3
  vert2 : Inport  Port=4
  vert3 : Inport  Port=5
  dA : Inport  Port=6
  ntri : Inport  Port=7
  normal : Inport  Port=8
  A_wave : Inport  Port=9
  k_wave : Inport  Port=10
  w_wave : Inport  Port=11
  rho : Inport  Port=12
  g : Inport  Port=13
  vert4 : Inport  Port=14
  vert5 : Inport  Port=15
  vert6 : Inport  Port=16
  dA1 : Inport  Port=17
  ntri1 : Inport  Port=18
  Zb : Inport  Port=19
  EAX : Inport  Port=20
  dX : Inport  Port=21
  Root_o : Inport  Port=22
  Add1 : Sum
  CG : Constant  Value=[32.3114; 0; 0;]
  MATLAB Function1 : MATLAB Function  TreatAsAtomicUnit=on
  MATLAB Function4 : MATLAB Function  TreatAsAtomicUnit=on
  Mux1 : Mux  Inputs=6
  Mux2 : Mux  Inputs=6
  Out1 : Outport
  wires:
  ntri1/1 -> MATLAB Function1/7(ntri)
  dA1/1 -> MATLAB Function1/6(dA)
  vert6/1 -> MATLAB Function1/5(vert3)
  vert5/1 -> MATLAB Function1/4(vert2)
  vert4/1 -> MATLAB Function1/3(vert1)
  Zb/1 -> MATLAB Function4/13(Zb), MATLAB Function1/13(Zb)
  vert2/1 -> MATLAB Function4/4(vert2)
  ntri/1 -> MATLAB Function4/7(ntri)
  normal/1 -> ?
  time/1 -> MATLAB Function4/1(time), MATLAB Function1/1(time)
  vert1/1 -> MATLAB Function4/3(vert1)
  Mux1/1 -> Add1/2
  vert3/1 -> MATLAB Function4/5(vert3)
  Mux2/1 -> Add1/1
  MATLAB Function4/2(Fy_total) -> Mux2/2
  MATLAB Function4/6(Mz_total) -> Mux2/6
  g/1 -> MATLAB Function4/12(g), MATLAB Function1/12(g)
  k_wave/1 -> MATLAB Function4/9(k_wave), MATLAB Function1/9(k_wave)
  dA/1 -> MATLAB Function4/6(dA)
  MATLAB Function4/5(My_total) -> Mux2/5
  MATLAB Function1/3(Fz_total) -> Mux1/3
  Add1/1 -> Out1/1
  MATLAB Function1/1(Fx_total) -> Mux1/1
  MATLAB Function4/1(Fx_total) -> Mux2/1
  MATLAB Function1/4(Mx_total) -> Mux1/4
  A_wave/1 -> MATLAB Function4/8(A_wave), MATLAB Function1/8(A_wave)
  rho/1 -> MATLAB Function4/11(rho), MATLAB Function1/11(rho)
  Xearth/1 -> MATLAB Function4/2(Xearth), MATLAB Function1/2(Xearth)
  MATLAB Function1/2(Fy_total) -> Mux1/2
  w_wave/1 -> MATLAB Function4/10(w_wave), MATLAB Function1/10(w_wave)
  MATLAB Function4/4(Mx_total) -> Mux2/4
  MATLAB Function4/3(Fz_total) -> Mux2/3
  EAX/1 -> MATLAB Function4/14(EAX), MATLAB Function1/14(EAX)
  dX/1 -> MATLAB Function4/15(dX), MATLAB Function1/15(dX)
  Root_o/1 -> MATLAB Function4/16(origin), MATLAB Function1/16(origin)
  CG/1 -> MATLAB Function4/17(xcg), MATLAB Function1/17(xcg)
  MATLAB Function1/5(My_total) -> Mux1/5
  MATLAB Function1/6(Mz_total) -> Mux1/6

== system Model_6DOF_dk/HDM/HDM B3/Wave, Virtual Mass and Hydrostatic/Wave Particle Motions/Hydrostatic Forces and Moments/X3 ==
  time : Inport
  Xearth : Inport  Port=2
  vert1 : Inport  Port=3
  vert2 : Inport  Port=4
  vert3 : Inport  Port=5
  dA : Inport  Port=6
  ntri : Inport  Port=7
  A_wave : Inport  Port=8
  k_wave : Inport  Port=9
  w_wave : Inport  Port=10
  rho : Inport  Port=11
  g : Inport  Port=12
  vert4 : Inport  Port=13
  vert5 : Inport  Port=14
  vert6 : Inport  Port=15
  dA1 : Inport  Port=16
  ntri1 : Inport  Port=17
  Zb : Inport  Port=18
  EAX : Inport  Port=19
  dX : Inport  Port=20
  Root_o : Inport  Port=21
  Add1 : Sum
  CG : Constant  Value=[32.3114; 0; 0;]
  MATLAB Function1 : MATLAB Function  TreatAsAtomicUnit=on
  MATLAB Function4 : MATLAB Function  TreatAsAtomicUnit=on
  Mux1 : Mux  Inputs=6
  Mux2 : Mux  Inputs=6
  Out1 : Outport
  wires:
  MATLAB Function1/6(Mz_total) -> Mux1/6
  MATLAB Function1/5(My_total) -> Mux1/5
  CG/1 -> MATLAB Function1/17(xcg), MATLAB Function4/17(xcg)
  Root_o/1 -> MATLAB Function1/16(origin), MATLAB Function4/16(origin)
  dX/1 -> MATLAB Function1/15(dX), MATLAB Function4/15(dX)
  EAX/1 -> MATLAB Function1/14(EAX), MATLAB Function4/14(EAX)
  MATLAB Function4/3(Fz_total) -> Mux2/3
  MATLAB Function4/4(Mx_total) -> Mux2/4
  w_wave/1 -> MATLAB Function1/10(w_wave), MATLAB Function4/10(w_wave)
  MATLAB Function1/2(Fy_total) -> Mux1/2
  Xearth/1 -> MATLAB Function1/2(Xearth), MATLAB Function4/2(Xearth)
  rho/1 -> MATLAB Function1/11(rho), MATLAB Function4/11(rho)
  A_wave/1 -> MATLAB Function1/8(A_wave), MATLAB Function4/8(A_wave)
  MATLAB Function1/4(Mx_total) -> Mux1/4
  MATLAB Function4/1(Fx_total) -> Mux2/1
  MATLAB Function1/1(Fx_total) -> Mux1/1
  Add1/1 -> Out1/1
  MATLAB Function1/3(Fz_total) -> Mux1/3
  MATLAB Function4/5(My_total) -> Mux2/5
  dA/1 -> MATLAB Function4/6(dA)
  k_wave/1 -> MATLAB Function1/9(k_wave), MATLAB Function4/9(k_wave)
  g/1 -> MATLAB Function1/12(g), MATLAB Function4/12(g)
  MATLAB Function4/6(Mz_total) -> Mux2/6
  MATLAB Function4/2(Fy_total) -> Mux2/2
  Mux2/1 -> Add1/1
  vert3/1 -> MATLAB Function4/5(vert3)
  Mux1/1 -> Add1/2
  vert1/1 -> MATLAB Function4/3(vert1)
  time/1 -> MATLAB Function1/1(time), MATLAB Function4/1(time)
  ntri/1 -> MATLAB Function4/7(ntri)
  vert2/1 -> MATLAB Function4/4(vert2)
  Zb/1 -> MATLAB Function1/13(Zb), MATLAB Function4/13(Zb)
  vert4/1 -> MATLAB Function1/3(vert1)
  vert5/1 -> MATLAB Function1/4(vert2)
  vert6/1 -> MATLAB Function1/5(vert3)
  dA1/1 -> MATLAB Function1/6(dA)
  ntri1/1 -> MATLAB Function1/7(ntri)

== system Model_6DOF_dk/HDM/HDM B3/Wave, Virtual Mass and Hydrostatic/Wave Particle Motions/Hydrostatic Forces and Moments/X4 ==
  time : Inport
  Xearth : Inport  Port=2
  vert1 : Inport  Port=3
  vert2 : Inport  Port=4
  vert3 : Inport  Port=5
  dA : Inport  Port=6
  ntri : Inport  Port=7
  normal : Inport  Port=8
  A_wave : Inport  Port=9
  k_wave : Inport  Port=10
  w_wave : Inport  Port=11
  rho : Inport  Port=12
  g : Inport  Port=13
  vert4 : Inport  Port=14
  vert5 : Inport  Port=15
  vert6 : Inport  Port=16
  dA1 : Inport  Port=17
  ntri1 : Inport  Port=18
  Zb : Inport  Port=19
  EAX : Inport  Port=20
  dX : Inport  Port=21
  Root_o : Inport  Port=22
  Add1 : Sum
  CG : Constant  Value=[32.3114; 0; 0;]
  MATLAB Function1 : MATLAB Function  TreatAsAtomicUnit=on
  MATLAB Function4 : MATLAB Function  TreatAsAtomicUnit=on
  Mux1 : Mux  Inputs=6
  Mux2 : Mux  Inputs=6
  Out1 : Outport
  wires:
  ntri1/1 -> MATLAB Function1/7(ntri)
  dA1/1 -> MATLAB Function1/6(dA)
  vert6/1 -> MATLAB Function1/5(vert3)
  vert5/1 -> MATLAB Function1/4(vert2)
  vert4/1 -> MATLAB Function1/3(vert1)
  Zb/1 -> MATLAB Function4/13(Zb), MATLAB Function1/13(Zb)
  vert2/1 -> MATLAB Function4/4(vert2)
  ntri/1 -> MATLAB Function4/7(ntri)
  normal/1 -> ?
  time/1 -> MATLAB Function4/1(time), MATLAB Function1/1(time)
  vert1/1 -> MATLAB Function4/3(vert1)
  Mux1/1 -> Add1/2
  vert3/1 -> MATLAB Function4/5(vert3)
  Mux2/1 -> Add1/1
  MATLAB Function4/2(Fy_total) -> Mux2/2
  MATLAB Function4/6(Mz_total) -> Mux2/6
  g/1 -> MATLAB Function4/12(g), MATLAB Function1/12(g)
  k_wave/1 -> MATLAB Function4/9(k_wave), MATLAB Function1/9(k_wave)
  dA/1 -> MATLAB Function4/6(dA)
  MATLAB Function4/5(My_total) -> Mux2/5
  MATLAB Function1/3(Fz_total) -> Mux1/3
  Add1/1 -> Out1/1
  MATLAB Function1/1(Fx_total) -> Mux1/1
  MATLAB Function4/1(Fx_total) -> Mux2/1
  MATLAB Function1/4(Mx_total) -> Mux1/4
  A_wave/1 -> MATLAB Function4/8(A_wave), MATLAB Function1/8(A_wave)
  rho/1 -> MATLAB Function1/11(rho), MATLAB Function4/11(rho)
  Xearth/1 -> MATLAB Function4/2(Xearth), MATLAB Function1/2(Xearth)
  MATLAB Function1/2(Fy_total) -> Mux1/2
  w_wave/1 -> MATLAB Function4/10(w_wave), MATLAB Function1/10(w_wave)
  MATLAB Function4/4(Mx_total) -> Mux2/4
  MATLAB Function4/3(Fz_total) -> Mux2/3
  EAX/1 -> MATLAB Function4/14(EAX), MATLAB Function1/14(EAX)
  dX/1 -> MATLAB Function4/15(dX), MATLAB Function1/15(dX)
  Root_o/1 -> MATLAB Function4/16(origin), MATLAB Function1/16(origin)
  CG/1 -> MATLAB Function4/17(xcg), MATLAB Function1/17(xcg)
  MATLAB Function1/5(My_total) -> Mux1/5
  MATLAB Function1/6(Mz_total) -> Mux1/6

== system Model_6DOF_dk/HDM/HDM B3/Wave, Virtual Mass and Hydrostatic/Wave Particle Motions/Hydrostatic Forces and Moments/XB ==
  time : Inport
  Xearth : Inport  Port=2
  vert1 : Inport  Port=3
  vert2 : Inport  Port=4
  vert3 : Inport  Port=5
  dA : Inport  Port=6
  ntri : Inport  Port=7
  normal : Inport  Port=8
  A_wave : Inport  Port=9
  k_wave : Inport  Port=10
  w_wave : Inport  Port=11
  rho : Inport  Port=12
  g : Inport  Port=13
  vert4 : Inport  Port=14
  vert5 : Inport  Port=15
  vert6 : Inport  Port=16
  dA1 : Inport  Port=17
  ntri1 : Inport  Port=18
  normal1 : Inport  Port=19
  Zb : Inport  Port=20
  EAX : Inport  Port=21
  dX : Inport  Port=22
  Root_o : Inport  Port=23
  Add1 : Sum
  CG : Constant  Value=[32.3114; 0; 0;]
  MATLAB Function1 : MATLAB Function  TreatAsAtomicUnit=on
  MATLAB Function4 : MATLAB Function  TreatAsAtomicUnit=on
  Mux1 : Mux  Inputs=6
  Mux2 : Mux  Inputs=6
  Out1 : Outport
  wires:
  normal1/1 -> ?
  ntri1/1 -> MATLAB Function1/7(ntri)
  dA1/1 -> MATLAB Function1/6(dA)
  vert6/1 -> MATLAB Function1/5(vert3)
  vert5/1 -> MATLAB Function1/4(vert2)
  vert4/1 -> MATLAB Function1/3(vert1)
  Zb/1 -> MATLAB Function4/13(Zb), MATLAB Function1/13(Zb)
  vert2/1 -> MATLAB Function4/4(vert2)
  ntri/1 -> MATLAB Function4/7(ntri)
  normal/1 -> ?
  time/1 -> MATLAB Function4/1(time), MATLAB Function1/1(time)
  vert1/1 -> MATLAB Function4/3(vert1)
  Mux1/1 -> Add1/2
  vert3/1 -> MATLAB Function4/5(vert3)
  Mux2/1 -> Add1/1
  MATLAB Function4/2(Fy_total) -> Mux2/2
  MATLAB Function4/6(Mz_total) -> Mux2/6
  g/1 -> MATLAB Function4/12(g), MATLAB Function1/12(g)
  k_wave/1 -> MATLAB Function4/9(k_wave), MATLAB Function1/9(k_wave)
  dA/1 -> MATLAB Function4/6(dA)
  MATLAB Function4/5(My_total) -> Mux2/5
  MATLAB Function1/3(Fz_total) -> Mux1/3
  Add1/1 -> Out1/1
  MATLAB Function1/1(Fx_total) -> Mux1/1
  MATLAB Function4/1(Fx_total) -> Mux2/1
  MATLAB Function1/4(Mx_total) -> Mux1/4
  A_wave/1 -> MATLAB Function4/8(A_wave), MATLAB Function1/8(A_wave)
  rho/1 -> MATLAB Function4/11(rho), MATLAB Function1/11(rho)
  Xearth/1 -> MATLAB Function4/2(Xearth), MATLAB Function1/2(Xearth)
  MATLAB Function1/2(Fy_total) -> Mux1/2
  w_wave/1 -> MATLAB Function4/10(w_wave), MATLAB Function1/10(w_wave)
  MATLAB Function4/4(Mx_total) -> Mux2/4
  MATLAB Function4/3(Fz_total) -> Mux2/3
  EAX/1 -> MATLAB Function4/14(EAX), MATLAB Function1/14(EAX)
  dX/1 -> MATLAB Function4/15(dX), MATLAB Function1/15(dX)
  Root_o/1 -> MATLAB Function4/16(origin), MATLAB Function1/16(origin)
  CG/1 -> MATLAB Function4/17(xcg), MATLAB Function1/17(xcg)
  MATLAB Function1/5(My_total) -> Mux1/5
  MATLAB Function1/6(Mz_total) -> Mux1/6

== matlab function Model_6DOF_dk/Controller/Marin PID ==
  settings: updateMethod=DISCRETE
  data: z_ref input; psi_ref input; Bv input; Bx input; dX output; Ts parameter
function dX   = fcn(z_ref,psi_ref,Bv,Bx,Ts)

persistent zerr_prev zerr_int_prev thetaerr_prev thetaerr_int_prev psierr_prev psierr_int_prev

%% Initialize
if isempty(zerr_prev)
        zerr_prev = 0;
        zerr_int_prev = 0;
        thetaerr_prev = 0;
        thetaerr_int_prev = 0;
        psierr_prev = 0;
        psierr_int_prev = 0;
end


%% Variables for feedback
x = Bx(1); y = Bx(2); z = Bx(3); phi = Bx(4); theta = Bx(5); psi = Bx(6);
p = [x;y;z];
uN = Bv(1); vN = Bv(2); wN = Bv(3); pB = Bv(4); qB=Bv(5); rB = Bv(6);
uB = -uN; vB = -vN; wB = wN;


%% Gains
KP_APz = 3;
KI_APz = 0*0.1044;
KD_APz = 3;

KP_APtheta = 3;
KI_APtheta = 0*0.1466;
KD_APtheta = 3;

KP_APpsi = 3;
KI_APpsi = 0;
KD_APpsi = 12.199;








%% Autopilot (depth)
zerr = z_ref - z;
zerrint = zerr*Ts+zerr_int_prev;
zerrdot = (zerr-zerr_prev)/Ts;
dvz = KP_APz*zerr+KI_APz*zerrint+KD_APz*zerrdot;

theta_ref = 0;
thetaerr = (theta_ref - theta)*180/pi;
thetaerrint = thetaerr*Ts+thetaerr_int_prev;
thetaerrdot = (thetaerr-thetaerr_prev)/Ts;
dvtheta = KP_APtheta*thetaerr+KI_APtheta*thetaerrint+KD_APtheta*thetaerrdot;

dv = dvz + dvtheta;

%% Autopilot (yaw)
psierr = (psi_ref - psi)*180/pi;
psierrint = psierr*Ts+psierr_int_prev;
psierrdot = (psierr-psierr_prev)/Ts;
dh = KP_APpsi*psierr+KI_APpsi*psierrint+KD_APpsi*psierrdot;


%% Control Allocation
d1 = -dv+dh; 
d2 = -dv-dh; 
d3 = dv-dh; 
d4 = dv+dh; 
d5 = dv; 
dX = [d1 ; d2 ; d3 ; d4 ; d5];





%% Save variables for next loop
zerr_prev = zerr;
zerr_int_prev = zerrint;
thetaerr_prev = thetaerr;
thetaerr_int_prev = thetaerrint;
psierr_prev = psierr;
psierr_int_prev = psierrint;

== matlab function Model_6DOF_dk/Controller/FF velocity ctrl ==
  settings: updateMethod=DISCRETE
  data: v_ref input; Bv input; Bx input; Ts parameter; n output
function n   = fcn(v_ref,Bv,Bx,Ts)


%% Variables for feedback
x = Bx(1); y = Bx(2); z = Bx(3); phi = Bx(4); theta = Bx(5); psi = Bx(6);
p = [x;y;z];
uN = Bv(1); vN = Bv(2); wN = Bv(3); pB = Bv(4); qB=Bv(5); rB = Bv(6);
uB = -uN; vB = -vN; wB = wN;

KP_n = 5;
FF_inv = 4;



%% Prop
n = -v_ref/FF_inv;

== matlab function Model_6DOF_dk/Controller/l1 aug - heading ==
  settings: updateMethod=DISCRETE
  data: y_ref input; Bv input; Bx input; y_aug output; Ts parameter; adap parameter; L1 parameter
function y_aug    = fcn(y_ref,Bv,Bx,Ts,adap,L1)
%pd,NomegaNI,

persistent xu xd


%% Variables for feedback
x = Bx(1); y = Bx(2); z = Bx(3); phi = Bx(4); theta = Bx(5); psi = Bx(6);
p = [x;y;z];
uN = Bv(1); vN = Bv(2); wN = Bv(3); pB = Bv(4); qB=Bv(5); rB = Bv(6);
uB = -uN; vB = -vN; wB = wN;

%% Control Parameters  
% Gains for PF augmentation
Ts = Ts;
Am = L1.Amz; Bm = L1.Bmz; Cm = L1.Cmz; 
Phiinv = L1.Phiinvz; Lambda = L1.Lambdaz;
Ao = L1.Aoz; Bo = L1.Boz; Co = L1.Coz;

%% Output Definition
y = psi;;

%% Initialize
if isempty(xu)
        xu = zeros(length(Ao),1);
        xd = Cm'*inv(Cm*Cm')*y;
        xu_next = xu;
        xd_next = xd;
end



%% L1 Augmentation - dive

if adap 

    yd = Cm*xd;
    vec1    =   [eye(size(Bm,2)); zeros(size(Am,1)-size(Bm,2),size(Bm,2))];
    sigma = -Phiinv*expm(Lambda*(Am/Lambda)*Ts)*vec1*(yd-y);

    xu_next = expm(Ao*Ts)*xu + inv(Ao)*(expm(Ao*Ts)-eye(length(Bo)))*(Bo*expm(-Am*Ts)*sigma);
    Kg = -inv(Cm*inv(Am)*Bm);
    ud = Kg*y_ref - Co*xu;

    xd_next = expm(Am*Ts)*xd + inv(Am)*(expm(Am*Ts)-eye(length(Am)))*(Bm*ud + sigma);

    y_aug = ud;

else 

    y_aug = y_ref;

    xd_next = xd;
    xu_next = xu;

end




%% Save variables for next loop
xu = xu_next;
xd = xd_next;

== matlab function Model_6DOF_dk/HDM/HDM B3/Effective Veloicity Calclation/MATLAB Function ==
  data: nh input; n1 input; aX output; n2 input; n3 input; n4 input; nB input; urX1 input; urX2 input; urX3 input; urX4 input; urXB input; UeX output
function [aX,UeX] = fcn(nh,n1,n2,n3,n4,nB,urX1,urX2,urX3,urX4,urXB)

%urXi: relative velocity of rigid body motion and wave particle velocity to the ith stern plane
%ni  : base vector of i-th plane's axis direction
%nh  : base vector of the hull axis direction
IP=zeros(5,1); %IP determines the sign of the angle of attack. if the dot product is negative, angle is greater than 90degs.
aX=zeros(5,1);

np1=dot(nh,urX1)*nh+dot(n1,urX1)*n1;
np2=dot(nh,urX2)*nh+dot(n2,urX2)*n2;
np3=dot(nh,urX3)*nh+dot(n3,urX3)*n3;
np4=dot(nh,urX4)*nh+dot(n4,urX4)*n4;
npB=dot(nh,urXB)*nh+dot(nB,urXB)*nB;

arg1=dot(np1,urX1)/(norm(np1)*norm(urX1));
arg2=dot(np2,urX2)/(norm(np2)*norm(urX2));
arg3=dot(np3,urX3)/(norm(np3)*norm(urX3));
arg4=dot(np4,urX4)/(norm(np4)*norm(urX4));
arg5=dot(npB,urXB)/(norm(npB)*norm(urXB));

%to prevent numerical error: acos returns complex solution. used if statement
if arg1 >=1
   aX(1,1)=0;
else
   aX(1,1)=acos(arg1)*180/pi*sqrt(2);
end

if arg2 >=1
   aX(2,1)=0;
else
   aX(2,1)=acos(arg2)*180/pi*sqrt(2);
end

if arg3 >=1
   aX(3,1)=0;
else
   aX(3,1)=acos(arg3)*180/pi*sqrt(2);
end

if arg4 >=1
   aX(4,1)=0;
else
   aX(4,1)=acos(arg4)*180/pi*sqrt(2);
end

if arg5 >=1
   aX(5,1)=0;
else
   aX(5,1)=acos(arg5)*180/pi;
end

d1=cross(n1,nh);
d2=cross(n2,nh);
d3=cross(n3,nh);
d4=cross(n4,nh);
dB=cross(nB,nh);

IP(1,1)=dot(d1,urX1);
IP(2,1)=dot(d2,urX2);
IP(3,1)=dot(d3,urX3);
IP(4,1)=dot(d4,urX4);
IP(5,1)=dot(dB,urXB);

for i=1:5
    if IP(i,1)<0
        aX(i,1)=-aX(i,1)
    end
end    

UeX=[norm(urX1); norm(urX2); norm(urX3); norm(urX4); norm(urXB);];
end
